simulink model "ADCS_onOrbit"  (R2024b)
settings: Solver=ode4  StartTime=0.0  StopTime=tspan  FixedStep=1  RelTol=1e-5
values from neighbouring files (symbols this model uses):
  A_list = [10*30; 10*30; 10*10; 10*30; 10*30; 10*10] * 1e-04    [acsLoadParameters.m]
  A_m = eye(3)    [acsLoadParameters.m]
  A_w = eye(3)    [acsLoadParameters.m]
  CD = 2.3    [acsLoadParameters.m]
  COP = [xAxis/2   0          0 ... (first row only)    [acsLoadParameters.m]
  dYear = decyear(YYYY,MM,DD)    [acsLoadParameters.m]
  e = 6.91944e-15    [acsLoadParameters.m]
  eta = 0.3    [acsLoadParameters.m]
  inc = 97.4377    [acsLoadParameters.m]
  J_body = [I_x 0 0; 0 I_y 0; 0 0 I_z]    [acsLoadParameters.m]
  J_wheels = [12894 0 0; 0 12774 0; 0 0 18389] * 1e-09    [acsLoadParameters.m]
  JD0 = juliandate(YYYY,MM,DD,HH,MIN,SEC)    [acsLoadParameters.m]
  K_d = 0.008    [acsLoadParameters.m]
  K_p = 0.003    [acsLoadParameters.m]
  K_w = 50e4    (= 500000)    [acsLoadParameters.m]
  m = 4    [acsLoadParameters.m]
  mag_moment = [0.005; 0.005; 0.005]    [acsLoadParameters.m]
  mu = 398600.4418    [acsLoadParameters.m]
  n_list = [1 0 0; 0 1 0; 0 0 1; -1 0 0; 0 -1 0; 0 0 -1]    [acsLoadParameters.m]
  omega = 0    [acsLoadParameters.m]    (also in orbit_plot_sfcn.m = block.InputPort(4).Data(:))
  p = 0.00000451    (= 4.51e-06)    [acsLoadParameters.m]    (also in cubesat_attitude_sfcn.m = ud.cubePos)
  P_0 = 0.0000001 * eye(7)    [acsLoadParameters.m]
  period = sqrt((4* pi^2 * semimajor_axis^3)/(mu))    [acsLoadParameters.m]
  q_ini = [0; 0; 0; 1]    [acsLoadParameters.m]
  raan = 226.816    [acsLoadParameters.m]
  rE = 6378.14    [acsLoadParameters.m]
  semimajor_axis = rE + h_apogee    (= 6913.14)    [acsLoadParameters.m]
  sigma_B_b = 0.05 * [1; 1; 1]    [acsLoadParameters.m]
  sigma_drift = 0.05 * [1; 1; 1] * 0    [acsLoadParameters.m]
  sigma_n = (0.05) * [1; 1; 1] * 0    [acsLoadParameters.m]
  sigma_S_b = 0.05 * [1; 1; 1]    [acsLoadParameters.m]
  tau = 300    [ATT_EKF_DOT.m]    (also in acsLoadParameters.m)
  true_anomaly = 0.0994843    [acsLoadParameters.m]
  w_b_ini = [0; 0.1; 0.1]    [acsLoadParameters.m]
  w_bias_0 = 0.0001 * [1; 1; 1] * 0    [acsLoadParameters.m]
  w_w_ini = [0; 0; 0]    [acsLoadParameters.m]
  wE = [0 0 15.04*(pi/180)*(1/3600)]    [acsLoadParameters.m]
undefined symbols (not defined in the file or in its folder): WMM2020
libraries: simulink_extras x13, matrix_library x9, sharedtransform x7, aerolibgravity2 x1, aerolibutil x1
(part 3 of 3)

== matlab function ADCS_onOrbit/GNC/Navigation/Extended Kalman Filter/MATLAB Function2 ==
  data: u input; var_n_gyro input; var_bias input; dt input; tau input; sigma_b_B input; sigma_s_B input; P input; q_plus output; K output; bias_plus output; P_plus output
function [q_plus, K, bias_plus, P_plus] = ATT_EKF(u, var_n_gyro, var_bias, dt, tau, sigma_b_B, sigma_s_B, P)

coder.extrinsic('invChol_mex')

% Yazan Chihabi 2018
% Nimish Dhawan 2025

%---------------------------------------
% Input arguments
%---------------------------------------

% Priori Estimates
%---------------------------------------
% q_pre
% bias_pre

% Priori Covariance Estimate
%---------------------------------------
% P_pre

% Angular velocity
%---------------------------------------
% w_pre

% Current Measurements
%---------------------------------------
% qm_mes


%---------------------------------------
% Output Arguments
%---------------------------------------

% Posteriori State Estimates
%---------------------------------------
% q_plus
% bias_plus

% Posteriori Covariance Estimates
%---------------------------------------
% P_plus


%---------------------------------------
% Input Vector Assignation
%---------------------------------------

K = zeros(7,6);
q_plus = [0;0;0;0];
P_plus = zeros(7,7);
bias_plus = [0;0;0];

t = dt;


q_pre            = u(1:4);
q_triad          = u(5:8);
s_I              = u(9:11);
m_I              = u(12:14);
isEclipse_prev   = u(15);
isEclipse        = u(16);
s_B_mes          = u(17:19);
controlMode      = u(20);
m_B_mes          = u(21:23);
w_mes            = u(24:26);
dw               = u(27:29);
bias_pre         = u(30:32);

if isEclipse_prev == 1 && isEclipse == 0
    q_pre = q_triad;
end

P_pre = P;

w_pre = w_mes-bias_pre;

var_n = var_n_gyro;

var_b = sigma_b_B.^2;
var_s = sigma_s_B.^2;

var_b = var_b.*(10^1); % Tuning factors for sensor weight shifting
var_s = var_s.*(10^-3); % lower variance implies more reliability

v1 = [var_s' var_b'];
R = diag(v1);

v2 = [var_n(1), var_n(2), var_n(3), 2*var_bias(1)/tau, 2*var_bias(2)/tau, 2*var_bias(3)/tau];

Q = diag(v2);




%-----------------------------------------------------------------------  
% Propagation Phase
%----------------------------------------------------------------------- 

% State propagation with nonlinear model using a KMI algorithm (Kutta-Merson - a Fifth-Order Runge-Kutta)
%----------------------------------------------------------------------------------------------------------
state_pre = [q_pre;bias_pre];

K1 = ATT_EKF_DOT([state_pre;  w_pre])*t;
K2 = ATT_EKF_DOT([state_pre + K1/3;  w_pre])*t;
K3 = ATT_EKF_DOT([state_pre + (K1+K2)/6;  w_pre])*t;
K4 = ATT_EKF_DOT([state_pre + (K1+3*K3)/8;  w_pre])*t;
K5 = ATT_EKF_DOT([state_pre + (K1+4*K4-3*K3)/2; w_pre])*t;

  state_minus  	= state_pre+(K1+4*K4+K5)/6;
  
  q_minus 		= state_minus(1:4)/norm(state_minus(1:4));
  bias_minus    = state_minus(5:7);

if  abs(dw(1))<0.01 && abs(dw(2))<0.01 && abs(dw(3))<0.01  && controlMode ~=4 % && isEclipse == 0
    %-------------------------------------------------------------------
    % Covariance Matrix Propagation
    q1 = q_minus(1); q2 = q_minus(2); q3 = q_minus(3); q4 = q_minus(4);
    wx = w_pre(1); wy = w_pre(2); wz = w_pre(3);

    w_skew = [0 -wz wy; wz 0 -wx; -wy wx 0];

    box_q = [q4 -q3 q2; q3 q4 -q1; -q2 q1 q4; -q1 -q2 -q3];

    omega_w = [-w_skew w_pre; -w_pre' 0];
    % State Matrix

    F = [0.5*omega_w, -0.5*box_q; zeros(3,4) , -1/tau*ones(3,3)];

    M = zeros(3,3); %gyro alignment matrix



     phi          	= (F*t)*(((F*t)/2)*(((F*t)/3)*((F*t)/4 + eye(7,7))+eye(7,7))+eye(7,7))+eye(7,7);
    G = [ -0.5*box_q, zeros(4,3); zeros(3,3), eye(3,3)];


    P_minus = F*P_pre*F' + G*Q*G';


    %-----------------------------------------------------------------------  
    % Correction Phase
    %----------------------------------------------------------------------- 

    % Reduced state representation
    state_minus = [q_minus(1:3); bias_minus];

    % Linearized measurement model
    q1 = q_minus(1); q2 = q_minus(2); q3 = q_minus(3); q4 = q_minus(4);
    ep = [q1; q2; q3];
    ep_skew = [0 -q3 q2; q3 0 -q1; -q2 q1 0];

    A = (q4.^2 - ep'*ep)*eye(3,3) + 2*ep*ep' - 2*q4*ep_skew;
    m_B = A*m_I;
    s_B = A*s_I;
    % H = [2*(A*m_B)' 0 0 0];

    m_x = m_I(1); m_y = m_I(2); m_z = m_I(3); 
    H1 = [ 2*m_x*q1 + 2*m_y*q2 + 2*m_z*q3, 2*m_y*q1 - 2*m_x*q2 - 2*m_z*q4, 2*m_y*q4 - 2*m_x*q3 + 2*m_z*q1, 2*m_x*q4 + 2*m_y*q3 - 2*m_z*q2;
     2*m_x*q2 - 2*m_y*q1 + 2*m_z*q4, 2*m_x*q1 + 2*m_y*q2 + 2*m_z*q3, 2*m_z*q2 - 2*m_y*q3 - 2*m_x*q4, 2*m_y*q4 - 2*m_x*q3 + 2*m_z*q1;
     2*m_x*q3 - 2*m_y*q4 - 2*m_z*q1, 2*m_x*q4 + 2*m_y*q3 - 2*m_z*q2, 2*m_x*q1 + 2*m_y*q2 + 2*m_z*q3, 2*m_x*q2 - 2*m_y*q1 + 2*m_z*q4];
    s_x = s_I(1); s_y = s_I(2); s_z = s_I(3); 
    H2 = [ 2*s_x*q1 + 2*s_y*q2 + 2*s_z*q3, 2*s_y*q1 - 2*s_x*q2 - 2*s_z*q4, 2*s_y*q4 - 2*s_x*q3 + 2*s_z*q1, 2*s_x*q4 + 2*s_y*q3 - 2*s_z*q2;
     2*s_x*q2 - 2*s_y*q1 + 2*s_z*q4, 2*s_x*q1 + 2*s_y*q2 + 2*s_z*q3, 2*s_z*q2 - 2*s_y*q3 - 2*s_x*q4, 2*s_y*q4 - 2*s_x*q3 + 2*s_z*q1;
     2*s_x*q3 - 2*s_y*q4 - 2*s_z*q1, 2*s_x*q4 + 2*s_y*q3 - 2*s_z*q2, 2*s_x*q1 + 2*s_y*q2 + 2*s_z*q3, 2*s_x*q2 - 2*s_y*q1 + 2*s_z*q4];


    H = [H2 zeros(3,3); H1 zeros(3,3)];
    
    
    
    % Kalman Gain
    K = (P_minus*H')*invChol_mex(H*P_minus*H' + R); 

    % Measured outputs
    obs_mes = [s_B_mes; m_B_mes];

    % Estimated outputs
    obs_est = [s_B; m_B];

    % State Correction

    obs_mes_skew = [0 -obs_mes(3) obs_mes(2); obs_mes(3) 0 -obs_mes(1); -obs_mes(2) obs_mes(1) 0];

    delta_states = K*(obs_mes - obs_est);

    % delta_states = K*(obs_mes_skew*obs_est);

    % delta_q_plus = [delta_states(1:3); 1];
    % delta_bias_plus = delta_states(4:6);
    % 
    % dq1 = delta_q_plus(1); dq2 = delta_q_plus(2); dq3 = delta_q_plus(3); dq4 = delta_q_plus(4); 
    % dq = [dq4, dq3 -dq2, dq1; -dq3, dq4, dq1, dq2; dq2, -dq1, dq4, dq3; -dq1, -dq2, -dq3, dq4];
    % 
    % 
    % q_plus =  dq*q_minus/norm(dq*q_minus);

    delta_q = delta_states(1:4);
    delta_bias = delta_states(5:7);

    dq1 = delta_q(1); dq2 = delta_q(2); dq3 = delta_q(3); dq4 = delta_q(4); 
    dq = [dq4, dq3 -dq2, dq1; -dq3, dq4, dq1, dq2; dq2, -dq1, dq4, dq3; -dq1, -dq2, -dq3, dq4];

    q_plus    = q_minus + delta_q;
    % q_plus = q_minus + delta_q/norm(delta_q);
    % q_plus    = dq*q_minus/norm(dq*q_minus);
    bias_plus = bias_minus + delta_bias;


    % Covariance matrix correction

      P_plus       	= (eye(7,7) - K*H) * P_minus;


    
elseif isEclipse == 1 && controlMode == 4
    q_plus = q_minus;
    bias_plus = bias_minus;
    K = zeros(7,6);
    P_plus = 0.001*eye(7,7);
    
elseif isEclipse == 0 && controlMode == 4 
    q_plus = q_triad;
    bias_plus = bias_minus;
    K = zeros(7,6);
    P_plus = 0.00000000001*eye(7,7);
elseif isEclipse == 1 && abs(dw(1))>0.01 && abs(dw(2))>0.01 && abs(dw(3))>0.01  && controlMode ~=4
    q_plus = q_minus;
    bias_plus = bias_minus;
    K = zeros(7,6);
    P_plus = 0.0001*eye(7,7);
else
    q_plus = q_triad;
    bias_plus = bias_minus;
    K = zeros(7,6);
    P_plus = 0.0001*eye(7,7);
end
% end

K = K;
q_plus = q_plus;
P_plus = P_plus;
bias_plus = bias_plus;

end

== matlab function ADCS_onOrbit/SENS/Gyroscope/MATLAB Function ==
  data: bias input; biasDot output; noise input
function biasDot = fcn(bias, noise)

tau = 300;
bias_noise = noise*[1;1;1];

biasDot = -(1/tau) * bias + bias_noise;

== matlab function ADCS_onOrbit/RWP/Orbit Propagator/External/MATLAB Function ==
  data: t input; r_SI output; JD0 input
function r_SI = sun_vector(t, JD0)

    JD = JD0 + 1.157e-05*t;
    TUT = (JD-2451545)/36525;
    mean_long = 280.4606184 + 36000.77005361*TUT;
    mean_anom = 357.5277233 + 35999.0534*TUT;
    obliquity = 23.439291 - 0.0130042*TUT;
    lambda_e = mean_long + 1.914666471 * sind(mean_anom) + 0.019994643 * sind(2*mean_anom);
    r_sun_norm = (1.000140612 - 0.016708617 * cosd(mean_anom) + 0.019994643 * sind(2*mean_anom)) * 149597870.691; % km
    r_SI = r_sun_norm * [cosd(lambda_e); cosd(obliquity) * sind(lambda_e); sind(obliquity) * sind(lambda_e)];

end

== matlab function ADCS_onOrbit/RWP/Nonlinear Spacecraft/Subsystem/MATLAB Function ==
  data: rpy output; q input; roll output; pitch output; yaw output
function [rpy, roll, pitch, yaw] = fcn(q)

    x = q(1);
    y = q(2);
    z = q(3);
    w = q(4);

    % Roll
    sinr_cosp = 2 * (w*x + y*z);
    cosr_cosp = 1 - 2 * (x^2 + y^2);
    roll = atan2(sinr_cosp, cosr_cosp);

    % Pitch
    sinp = 2 * (w*y - z*x);
    sinp = max(min(sinp, 1), -1);
    pitch = asin(sinp);

    % Yaw
    siny_cosp = 2 * (w*z + x*y);
    cosy_cosp = 1 - 2 * (y^2 + z^2);
    yaw = atan2(siny_cosp, cosy_cosp);

    rpy = [roll; pitch; yaw];

    % output = unwrap(output);  % if working in degrees



end

== matlab function ADCS_onOrbit/RWP/Orbit Propagator/External/MATLAB Function1 ==
  data: r_S input; s output
function s = fcn(r_S)

s = r_S/norm(r_S);

== matlab function ADCS_onOrbit/GNC/Controller/Control Algorithm/MATLAB Function ==
  data: opMode input; t input; T_w output; period input; betaDot input; B_meas input; w input; w_skew input; J_body input; J_wheels input; K_p input; K_d input; K_w input; q_error input; w_error input; h_w input; M output; detumbleMode output
function [T_w, M, detumbleMode] = fcn(opMode ,t, period, betaDot, B_meas, w, w_skew, J_body, J_wheels, K_p, K_d, K_w, q_error, w_error, h_w)

T_w = [0; 0; 0];
M = [0; 0; 0];
Mx = M(1); My = M(2); Mz = M(3);
w_ref = deg2rad(0.2);
detumbleMode = 0;

% Modified PD control
if opMode ~= 4 && opMode ~= 5 && opMode ~= 6 && opMode ~= 7 && opMode ~= 8
    T_w = w_skew * J_body * w - K_p * eye(3) * q_error - K_d * eye(3) * w_error;

% B-dot 
elseif opMode == 8
    M = -K_w * cross(B_meas, w);

% No control
elseif opMode == 6 || opMode == 7
    T_w = [0; 0; 0];
    M = [0; 0; 0];

% Desaturation (incomplete)
elseif opMode == 5
    T_w = [0; 0; 0];
    M = [0; 0; 0];   

% Simple Bdot Detumble (works)
elseif opMode == 4
    if t < (1*period) && t > 200
        M = -K_w * cross(B_meas, w);
    elseif t > 1 * period && abs(norm(w)) < 0.05
        T_w = w_skew * J_body * w - K_p * eye(3) * q_error - K_d * eye(3) * w_error;
    else
        T_w = [0; 0; 0];
        M = [0; 0; 0]; 
    end

% Detumble Y-thompson mode (incomplete)
elseif opMode == 10
    if t < (1*period) && t > 200
        Kd = 3.5;
        My = Kd * betaDot;
        M = [0; My; 0];
        detumbleMode = 1;
    
    elseif t < (3*period) && t > (0.6*period)
        Kd = 7.5;
        Ks = 2.5;
        My = Kd * betaDot;
        if B_meas(3) > B_meas(1)
            Mx = Ks * (w(2)-w_ref) * sign(B_meas(3));
            Mz = 0;
        elseif B_meas(1) > B_meas(3)
            Mz = Ks * (w(2)-w_ref) * sign(B_meas(1));
            Mx = 0;
        end
    
        M = [Mx; My; Mz];
        T_w = [0; 0; 0];
        detumbleMode = 2;
    
    elseif t < (4*period) && t > (3*period)
        goalSpeed = w_ref * J_body(2,2) / J_wheels(3,3);
        
        Nwy = K_d * w(2) - K_p * q_error(2);
        T_w = [0; Nwy; 0];
    
        hwy = h_w(2);
        hwy_ref = goalSpeed * J_wheels(3,3);
        Kwy = 0;
    
        e = [K_d*w(1) + K_p*q_error(1);
         Kwy*(hwy - hwy_ref);
         K_d*w(3) + K_p*q_error(3)];
    
        M = cross(e, B_meas) / norm(B_meas);
        detumbleMode = 3;
    
    elseif t > (4*period) 
        T_w = w_skew * J_body * w - K_p * eye(3) * q_error - K_d * eye(3) * w_error;
        detumbleMode = 4;
    end
end

end

== matlab function ADCS_onOrbit/GNC/Controller/Control Algorithm/skew symmetric ==
  data: M input; skew output
function skew = skew_matrix(M)

    skew = [0 M(3) -M(2)
            -M(3) 0 M(1)
            M(2) -M(1) 0];

end

== matlab function ADCS_onOrbit/GNC/Controller/Control Algorithm/MATLAB Function3 ==
  data: By input; beta output; B input
function beta = fcn(By, B)

beta = acos(By / norm(B));

== matlab function ADCS_onOrbit/ACT/Wheels + Magnetorquers/Magnetorquer 1/skew symmetric ==
  data: M input; skew output
function skew = skew_matrix(M)

    skew = [0 M(3) -M(2)
            -M(3) 0 M(1)
            M(2) -M(1) 0];

end

== matlab function ADCS_onOrbit/ACT/Wheels + Magnetorquers/Magnetorquer 2/skew symmetric ==
  data: M input; skew output
function skew = skew_matrix(M)

    skew = [0 M(3) -M(2)
            -M(3) 0 M(1)
            M(2) -M(1) 0];

end

== matlab function ADCS_onOrbit/ACT/Wheels + Magnetorquers/Magnetorquer 3/skew symmetric ==
  data: M input; skew output
function skew = skew_matrix(M)

    skew = [0 M(3) -M(2)
            -M(3) 0 M(1)
            M(2) -M(1) 0];

end

== matlab function ADCS_onOrbit/ACT/Wheels + Magnetorquers/Wheel 1/MATLAB Function ==
  data: u input; y output
function y = fcn(u)

y = 1/u;

== matlab function ADCS_onOrbit/ACT/Wheels + Magnetorquers/Wheel 2/MATLAB Function ==
  data: u input; y output
function y = fcn(u)

y = 1/u;

== matlab function ADCS_onOrbit/RWP/Orbit Propagator/Internal/MATLAB Function1 ==
  data: t input; r_SI output; JD0 input
function r_SI = sun_vector(t, JD0)

    JD = JD0 + 1.157e-05*t;
    TUT = (JD-2451545)/36525;
    mean_long = 280.4606184 + 36000.77005361*TUT;
    mean_anom = 357.5277233 + 35999.0534*TUT;
    obliquity = 23.439291 - 0.0130042*TUT;
    lambda_e = mean_long + 1.914666471 * sind(mean_anom) + 0.019994643 * sind(2*mean_anom);
    r_sun_norm = (1.000140612 - 0.016708617 * cosd(mean_anom) + 0.019994643 * sind(2*mean_anom)) * 149597870.691; % km
    r_SI = r_sun_norm * [cosd(lambda_e); cosd(obliquity) * sind(lambda_e); sind(obliquity) * sind(lambda_e)];

end

== matlab function ADCS_onOrbit/RWP/Orbit Propagator/Internal/MATLAB Function2 ==
  data: r_S input; s output
function s = fcn(r_S)

s = r_S/norm(r_S);

== matlab function ADCS_onOrbit/SENS/Gyroscope/MATLAB Function1 ==
  data: w_sc input; w_meas output; bias input; noise input
function w_meas = fcn(w_sc, bias, noise)

rand_w = noise * [1; 1; 1];

w_bias_const = [0; 0; 0];

w_meas = w_sc + w_bias_const + bias + rand_w;

== matlab function ADCS_onOrbit/ACT/Wheels + Magnetorquers/Wheel 3/MATLAB Function ==
  data: u input; y output
function y = fcn(u)

y = 1/u;

== matlab function ADCS_onOrbit/RWP/Orbit Propagator/Internal/Orbit Elements/oe2rv ==
  data: a input; r_eci output; e input; i input; RAAN input; omega input; nu input; v_eci output; mu input
function [r_eci, v_eci] = oe2rv(a, e, i, RAAN, omega, nu, mu)

    % Step 1: Position & velocity in Perifocal (PQW) frame
    p = a * (1 - e^2);
    r_pqw = (p / (1 + e*cos(nu))) * [cos(nu); sin(nu); 0];
    v_pqw = sqrt(mu / p) * [-sin(nu); e + cos(nu); 0];

    % Step 2: Rotation matrices
    R3_W = [cos(RAAN) -sin(RAAN) 0; sin(RAAN) cos(RAAN) 0; 0 0 1];
    R1_i = [1 0 0; 0 cos(i) -sin(i); 0 sin(i) cos(i)];
    R3_w = [cos(omega) -sin(omega) 0; sin(omega) cos(omega) 0; 0 0 1];
    Q_pX = R3_W * R1_i * R3_w;

    % Step 3: Convert to ECI
    r_eci = Q_pX * r_pqw;
    v_eci = Q_pX * v_pqw;
end

== matlab function ADCS_onOrbit/RWP/Orbit Propagator/Internal/Two Body/MATLAB Function1 ==
  data: r_I input; a_I output; mu input
function a_I = fcn(r_I, mu)

a_I = r_I .* (-mu / (norm(r_I)^3));

end

== matlab function ADCS_onOrbit/RWP/Orbit Propagator/Internal/Two Body/MATLAB Function3 ==
  data: r input; a_j2 output; mu input; rE input
function a_j2 = J2_perturbation(r, mu, rE)

    J2 = 1.08263e-3;

    x = r(1); y = r(2); z = r(3);
    r_norm = norm(r);

    factor = -(3/2) * J2 * mu * rE^2 / r_norm^5;
    zx2_r2 = 5*z^2 / r_norm^2;

    a_j2 = factor * [
        x * (1 - zx2_r2);
        y * (1 - zx2_r2);
        z * (3 - zx2_r2)
    ];
end

== matlab function ADCS_onOrbit/ACT/Wheels + Magnetorquers/MATLAB Function1 ==
  data: M_c input; M_cmd output; rodsEnable input
function M_cmd = fcn(M_c, rodsEnable)

if rodsEnable == 1
    M_cmd = M_c;
else
    M_cmd = [0; 0; 0];
end

end

== matlab function ADCS_onOrbit/GNC/Navigation/Extended Kalman Filter/Subsystem/MATLAB Function ==
  data: rpy output; q input; roll output; pitch output; yaw output
function [rpy, roll, pitch, yaw] = fcn(q)

    x = q(1);
    y = q(2);
    z = q(3);
    w = q(4);

    % Roll
    sinr_cosp = 2 * (w*x + y*z);
    cosr_cosp = 1 - 2 * (x^2 + y^2);
    roll = atan2(sinr_cosp, cosr_cosp);

    % Pitch
    sinp = 2 * (w*y - z*x);
    sinp = max(min(sinp, 1), -1);
    pitch = asin(sinp);

    % Yaw
    siny_cosp = 2 * (w*z + x*y);
    cosy_cosp = 1 - 2 * (y^2 + z^2);
    yaw = atan2(siny_cosp, cosy_cosp);

    rpy = [roll; pitch; yaw];

    % output = unwrap(output);  % if working in degrees



end

== matlab function ADCS_onOrbit/GNC/Guidance/Target Pointing/MATLAB Function ==
  data: Re input; r_target_ecef output; target_lat input; target_lon input
function r_target_ecef = fcn(Re, target_lat, target_lon)

lat = deg2rad(target_lat);
lon = deg2rad(target_lon);

x_ecef = Re * cos(lat) * cos(lon);
y_ecef = Re * cos(lat) * sin(lon);
z_ecef = Re * sin(lat);

r_target_ecef = [x_ecef; y_ecef; z_ecef];

== matlab function ADCS_onOrbit/OBC/MATLAB Function ==
  data: internal input; mode output; fromTable input; wheelsEnable output; rodsEnable output
function [mode, wheelsEnable, rodsEnable] = fcn(internal, fromTable)

if internal ~= 2
    mode = internal;
    wheelsEnable = 1;
    rodsEnable = 1;
else
    mode = fromTable(1);
    wheelsEnable = fromTable(3);
    rodsEnable = fromTable(2);
end

end

== matlab function ADCS_onOrbit/RWP/Nonlinear Spacecraft/Spacecraft Dynamics/skew symmetric ==
  data: M input; skew output
function skew = skew_matrix(M)

    skew = [0 M(3) -M(2)
            -M(3) 0 M(1)
            M(2) -M(1) 0];

end
